simulink model "imc_conv_d"  (Simulink 5.0)
settings: Solver=ode45  StartTime=0.0  StopTime=10  RelTol=1e-3
values from neighbouring files (symbols this model uses):
  A = [1 -0.44]    [visc_imc1.m]
  B = [0.51 1.21]    [visc_imc1.m]
  R = conv(Bg,R)    [imc_stable.m]
  S = conv(Bf,A)    [imc_stable.m]
  Ts = 3    [lewin_imc1.m]    (also in lewin_imc_general.m; visc_imc1.m = 0.1)
undefined symbols (not defined in the file or in its folder): zk
settings Model: Creator=kannanm  LastModifiedBy=kannan  ExtModeAutoUpdateStatusClock=off

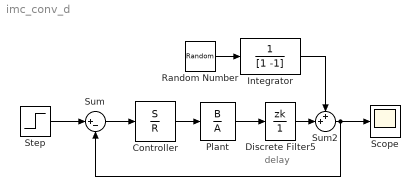
== system imc_conv_d ==
  note: delay
  Controller : DiscreteFilter  Numerator=S  Denominator=R  SampleTime=Ts
  Discrete Filter5 : DiscreteFilter  Numerator=zk  Denominator=1  SampleTime=Ts
  Integrator : DiscreteFilter  Numerator=1  Denominator=[1 -1]  SampleTime=Ts
  Plant : DiscreteFilter  Numerator=B  Denominator=A  SampleTime=Ts
  Random Number : RandomNumber  Variance=0.0  SampleTime=Ts
  Scope : Scope
      settings: YMin=-6e+164  YMax=1.02293e+149
  Step : Step  SampleTime=Ts
  Sum : Sum  Inputs=|+-  SaturateOnIntegerOverflow=on
  Sum2 : Sum  Inputs=++|  SaturateOnIntegerOverflow=on
  wires:
  Plant/1 -> Discrete Filter5/1
  Integrator/1 -> Sum2/1
  Sum2/1 -> Scope/1, Sum/2
  Discrete Filter5/1 -> Sum2/2
  Random Number/1 -> Integrator/1
  Sum/1 -> Controller/1
  Controller/1 -> Plant/1
  Step/1 -> Sum/1
